simulink model "Train_Model_Real"  (R2025b)
settings: Solver=VariableStepAuto  StartTime=0.0  StopTime=10.0  RelTol=1e-3
values from neighbouring files (symbols this model uses):
  A_d = sys_rd.A    [Working Model Draft.m]    (also in Working_Model_Draft.m; Working_Model_Final.m)
  B_d = sys_rd.B    [Working Model Draft.m]    (also in Working_Model_Draft.m; Working_Model_Final.m)
  C_d = sys_rd.C    [Working Model Draft.m]    (also in Working_Model_Draft.m; Working_Model_Final.m)
  K_d = dlqr(A_d, B_d, Q, R)    [Working Model Draft.m]    (also in Working_Model_Draft.m; Working_Model_Final.m)
  student_ID = 11540435    [Working Model Draft.m]    (also in Working_Model_Draft.m; Working_Model_Final.m)
  Ts = 1 / (20 * fastest_pole)    [Working Model Draft.m]    (also in Working_Model_Draft.m = 0.01; Working_Model_Final.m = 0.01)
  ustar = (ba1 + ba2) * vstar^2    (= 11728.3950617)    [Working Model Draft.m]    (also in Working_Model_Draft.m = 8979.55246914; Working_Model_Final.m = 9500)
  x0 = [Lc; 0; 0]    [Working Model Draft.m]    (also in Working_Model_Draft.m = [0.1; 87; 87]; Working_Model_Final.m = [0.1; vstar-perturb; vstar-perturb])
  z_hat0 = [Lc; vstar; vstar]    [Working Model Draft.m]    (also in Working_Model_Draft.m = [0.1; 0; 0]; Working_Model_Final.m = [0.1; vstar-perturb; vstar-perturb])
  zstar = [Lc; vstar; vstar]    [Working Model Draft.m]    (also in Working_Model_Draft.m = [0.1; vstar; vstar]; Working_Model_Final.m = [0; vstar; vstar])
undefined symbols (not defined in the file or in its folder): Discrete, Time
libraries: ctrlSharedLib x1, simulink x1
settings Model: Creator=froessil  LastModifiedBy=gamzf

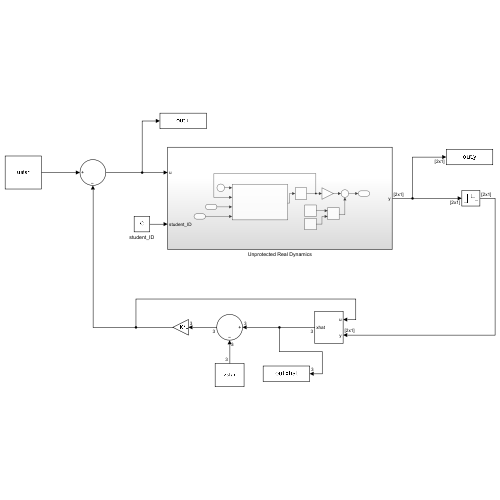
[thumbnail: Simulink's stored preview of the top-level diagram]
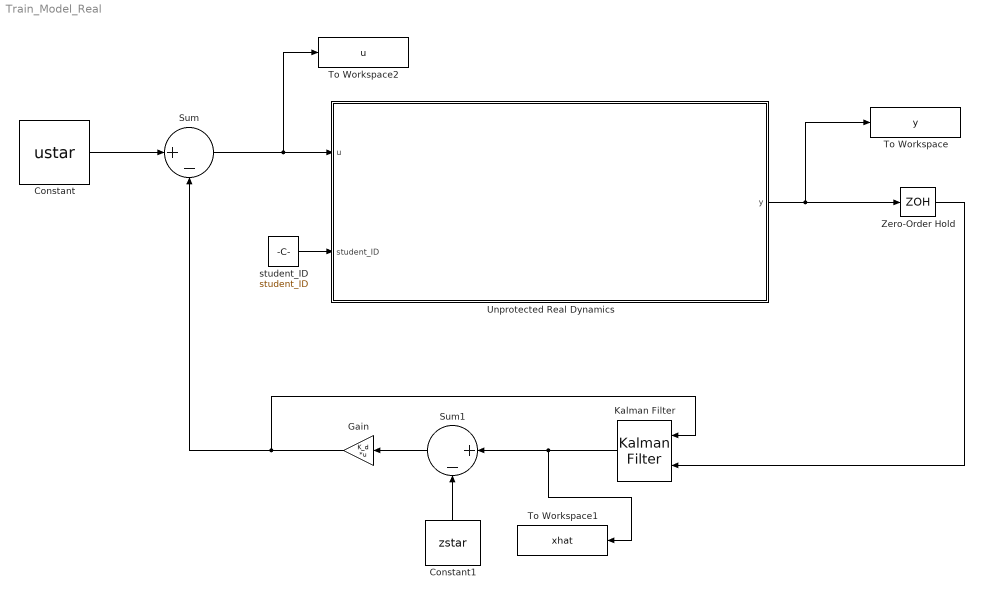
== system Train_Model_Real ==
  Constant : Constant  Value=ustar
  Constant1 : Constant  Value=zstar
  Gain : Gain  Gain=K_d  Multiplication=Matrix(K*u)
  Kalman Filter : ctrlSharedLib/Kalman Filter  TimeDomain=Discrete-Time  UseCurrentEstimator=on  ModelSource=LTI State-Space Variable  ModelSourceVariable=ss(A_d, B_d, C_d, zeros(2,1), Ts)  A=0.95  B=1  C=1  D=0  NumberOfStates=1  NumberOfInputs=1  NumberOfOutputs=1  InitialEstimateSource=Dialog  X0=z_hat0  P0=10  UseK=off  UseGH=off  NumberOfProcessNoiseInputs=1  G=1  TimeInvariantG=on  H=0  TimeInvariantH=on  Q=0.05  TimeInvariantQ=on  R=1  TimeInvariantR=on  N=0  TimeInvariantN=on  AddInputPort=on  AddEnablePort=off  OutputEstimatedY=off  OutputP=off  Ts=-1
  Sum : Sum  Inputs=|+-
  Sum1 : Sum  Inputs=|+-
  To Workspace : ToWorkspace  VariableName=y  SampleTime=-1
      settings: Save2DSignal=2-D array (concatenate along first dimension)
  To Workspace1 : ToWorkspace  VariableName=xhat  SampleTime=Ts
      settings: Save2DSignal=2-D array (concatenate along first dimension)
  To Workspace2 : ToWorkspace  VariableName=u  SampleTime=Ts
      settings: Save2DSignal=2-D array (concatenate along first dimension)
  Unprotected Real Dynamics : Subsystem
  Zero-Order Hold : ZeroOrderHold  SampleTime=Ts
  student_ID : Constant  Value=student_ID
  wires:
  student_ID/1 -> Unprotected Real Dynamics/2(student_ID)
  Kalman Filter/1 -> To Workspace1/1, Sum1/1
  Sum/1 -> To Workspace2/1, Unprotected Real Dynamics/1(u)
  Zero-Order Hold/1 -> Kalman Filter/2
  Unprotected Real Dynamics/1(y) -> To Workspace/1, Zero-Order Hold/1
  Constant/1 -> Sum/1
  Gain/1 -> Kalman Filter/1, Sum/2
  Sum1/1 -> Gain/1
  Constant1/1 -> Sum1/2

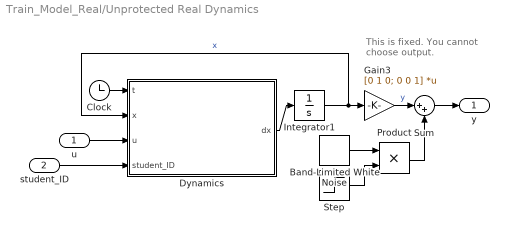
== system Train_Model_Real/Unprotected Real Dynamics ==
  note: This is fixed. You cannot choose output.
  u : Inport
  student_ID : Inport  Port=2
  Band-Limited White Noise : simulink/Sources/Band-Limited White Noise  Cov=[0.001]  Ts=Ts  seed=student_ID
  Clock : Clock
  "Dynamics " : MATLAB Function  TreatAsAtomicUnit=on
  Gain3 : Gain  Gain=[0 1 0; 0 0 1]  Multiplication=Matrix(K*u)
  Integrator1 : Integrator  InitialCondition=x0
  Product : Product
  Step : Step  Time=0  SampleTime=0
  Sum : Sum  Inputs=|++
  y : Outport
  wires:
  Integrator1/1 -> "Dynamics "/2(x), Gain3/1  "x"
  Clock/1 -> "Dynamics "/1(t)
  u/1 -> "Dynamics "/3(u)
  "Dynamics "/1(dx) -> Integrator1/1
  student_ID/1 -> "Dynamics "/4(student_ID)
  Gain3/1 -> Sum/1  "y"
  Sum/1 -> y/1
  Band-Limited White Noise/1 -> Product/1
  Product/1 -> Sum/2
  Step/1 -> Product/2

== matlab function Train_Model_Real/Unprotected Real Dynamics/Dynamics  ==
  data: t input; x input; u input; student_ID input; dx output
function dx = Train_Dynamics(t, x, u, student_ID)
dx = zeros(3,1);
dx = Train_Dynamics(t, x, u, student_ID);
